simulink model "SensorFaultInj"  (R2013a)
settings: Solver=FixedStepDiscrete  SolverMode=SingleTasking  StartTime=0.0  StopTime=SimLength  FixedStep=SampleTime  RelTol=1e-3
values from neighbouring files (symbols this model uses):
  GlobalSeed = 10    [start_framework07.m]
  SampleTime = 0.01    [start_framework07.m]
  SimLength = 40    [start_framework07.m]
undefined symbols (not defined in the file or in its folder): DiscIntNeverNeededParam
libraries: dspswit3 x48, simulink x32
(part 1 of 9)
settings Model: Creator=Maik  LastModifiedBy=Maik
settings DebuggingCC: AlgebraicLoopMsg=none  UnconnectedOutputMsg=none  BusObjectLabelMismatch=none

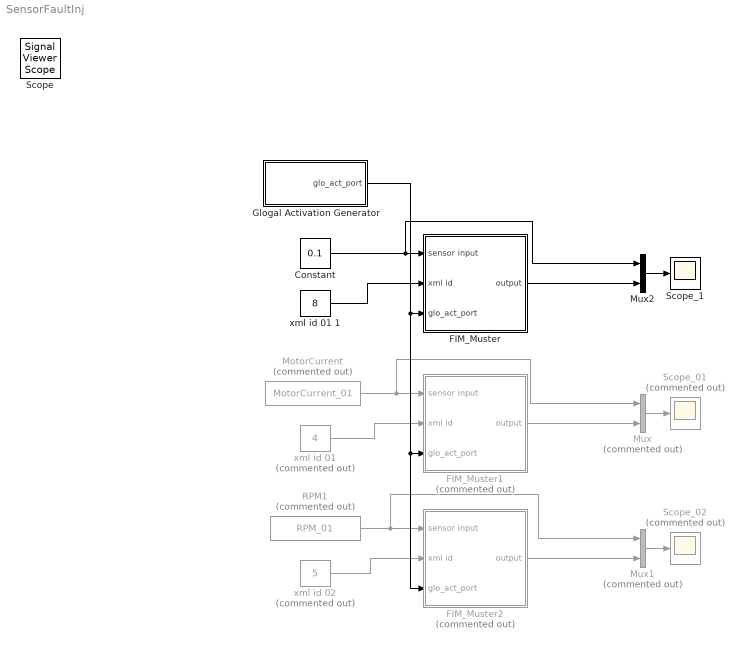
== system SensorFaultInj ==
  Constant : Constant  Value=0.1
  FIM_Muster : Subsystem
  FIM_Muster1 : Subsystem  Commented=on
  FIM_Muster2 : Subsystem  Commented=on
  Glogal Activation Generator : Subsystem  TreatAsAtomicUnit=on
  "MotorCurrent " : FromWorkspace  Commented=on  VariableName=MotorCurrent_01  SampleTime=SampleTime
  Mux : Mux  Commented=on  Inputs=2
  Mux1 : Mux  Commented=on  Inputs=2
  Mux2 : Mux  Inputs=2
  RPM1 : FromWorkspace  Commented=on  VariableName=RPM_01  SampleTime=SampleTime
  Scope_01 : Scope  Commented=on
      settings: YMin=0  YMax=4
  Scope_02 : Scope  Commented=on
      settings: YMin=0  YMax=20000
  Scope_1 : Scope
      settings: TimeRange=40  YMin=0.1  YMax=0.165  SaveName=SensordataEva01  MaxDataPoints=50000
  "xml id 01 " : Constant  Commented=on  Value=4  OutDataTypeStr=single
  xml id 01 1 : Constant  Value=8  OutDataTypeStr=single
  xml id 02 : Constant  Commented=on  Value=5  OutDataTypeStr=single
  Scope : SignalViewerScope  IOType=viewer  RefreshTime=0.035000
  wires:
  "MotorCurrent "/1 -> FIM_Muster1/1(sensor input), Mux/1
  "xml id 01 "/1 -> FIM_Muster1/2(xml id)
  Mux/1 -> Scope_01/1
  FIM_Muster1/1(output) -> Mux/2
  xml id 02/1 -> FIM_Muster2/2(xml id)
  Mux1/1 -> Scope_02/1
  FIM_Muster2/1(output) -> Mux1/2
  RPM1/1 -> FIM_Muster2/1(sensor input), Mux1/1
  Mux2/1 -> Scope_1/1
  FIM_Muster/1(output) -> Mux2/2
  Constant/1 -> Mux2/1, FIM_Muster/1(sensor input)
  xml id 01 1/1 -> FIM_Muster/2(xml id)
  Glogal Activation Generator/1(glo_act_port) -> FIM_Muster2/3(glo_act_port), FIM_Muster1/3(glo_act_port), FIM_Muster/3(glo_act_port)

== system SensorFaultInj/FIM_Muster ==
  sensor input : Inport
  xml id : Inport  Port=2
  glo_act_port : Inport  Port=3
  Fault Injection Modul : Subsystem
  Local Activation Generator : Subsystem
  Parser Modul : Subsystem
  logger : Subsystem
  output : Outport
  wires:
  Parser Modul/1(schedule_port) -> Local Activation Generator/1(schedule_port), Fault Injection Modul/2(schedule_port)
  Parser Modul/2(occurrnce_port) -> Local Activation Generator/2(occurrence_port)
  Local Activation Generator/1(activation_port) -> Fault Injection Modul/3(activation_port)
  Fault Injection Modul/1(Out1) -> logger/2("input "), output/1
  sensor input/1 -> Fault Injection Modul/1(sensor input)
  xml id/1 -> logger/1(xml_id), Parser Modul/1(xml id)
  Parser Modul/3(parameter_port) -> Local Activation Generator/3("param_port "), Fault Injection Modul/4(parameter_port)
  Fault Injection Modul/2("amplitude_port ") -> logger/4("amp_port ")
  Local Activation Generator/2(log_port) -> logger/3("act_port ")
  glo_act_port/1 -> Local Activation Generator/4(glo_act_port)

== system SensorFaultInj/FIM_Muster1 ==
  sensor input : Inport
  xml id : Inport  Port=2
  glo_act_port : Inport  Port=3
  Fault Injection Modul : Subsystem
  Parser Modul : Subsystem
  logger : Subsystem
  occurrence1 : Subsystem
  output : Outport
  wires:
  Parser Modul/1(schedule_port) -> occurrence1/1(schedule_port), Fault Injection Modul/2(schedule_port)
  Parser Modul/2(occurrnce_port) -> occurrence1/2(occurrence_port)
  occurrence1/1(activation_port) -> Fault Injection Modul/3(activation_port)
  Fault Injection Modul/1(Out1) -> logger/2("input "), output/1
  sensor input/1 -> Fault Injection Modul/1(sensor input)
  xml id/1 -> logger/1(xml_id), Parser Modul/1(xml id)
  Parser Modul/3(parameter_port) -> occurrence1/3("param_port "), Fault Injection Modul/4(parameter_port)
  Fault Injection Modul/2("amplitude_port ") -> logger/4("amp_port ")
  occurrence1/2(log_port) -> logger/3("act_port ")
  glo_act_port/1 -> occurrence1/4(glo_act_port)

== system SensorFaultInj/FIM_Muster2 ==
  sensor input : Inport
  xml id : Inport  Port=2
  glo_act_port : Inport  Port=3
  Fault Injection Modul : Subsystem
  Parser Modul : Subsystem
  logger : Subsystem
  occurrence1 : Subsystem
  output : Outport
  wires:
  Parser Modul/1(schedule_port) -> occurrence1/1(schedule_port), Fault Injection Modul/2(schedule_port)
  Parser Modul/2(occurrnce_port) -> occurrence1/2(occurrence_port)
  occurrence1/1(activation_port) -> Fault Injection Modul/3(activation_port)
  Fault Injection Modul/1(Out1) -> logger/2("input "), output/1
  sensor input/1 -> Fault Injection Modul/1(sensor input)
  xml id/1 -> logger/1(xml_id), Parser Modul/1(xml id)
  Parser Modul/3(parameter_port) -> occurrence1/3("param_port "), Fault Injection Modul/4(parameter_port)
  Fault Injection Modul/2("amplitude_port ") -> logger/4("amp_port ")
  occurrence1/2(log_port) -> logger/3("act_port ")
  glo_act_port/1 -> occurrence1/4(glo_act_port)

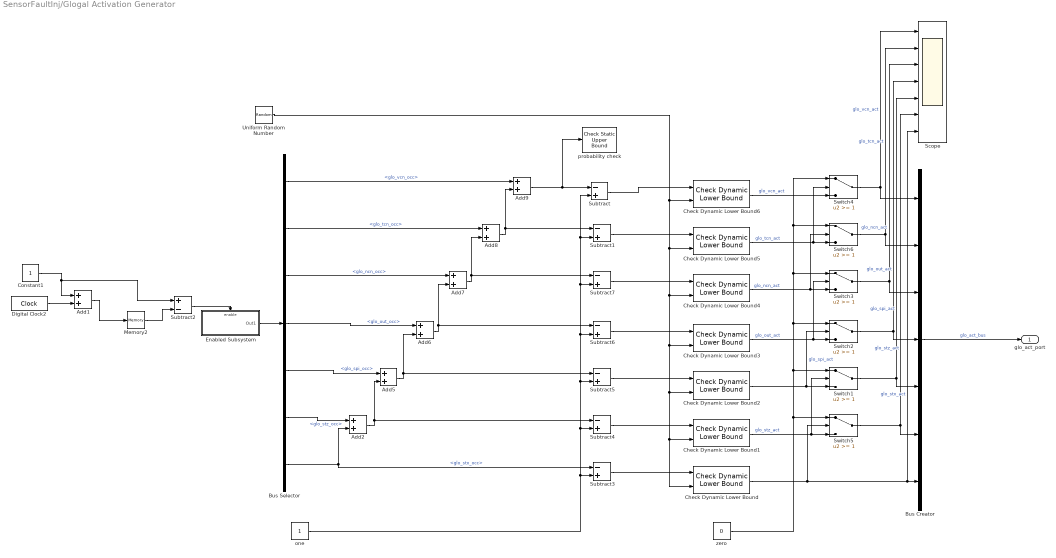
== system SensorFaultInj/Glogal Activation Generator ==
  Add{1..2,5..9} (7 alike) : Sum
  Bus Creator : BusCreator  Inputs=7
  Bus Selector : BusSelector  OutputSignals=glo_vcn_occ,glo_tcn_occ,glo_ncn_occ,glo_out_occ,glo_spi_occ,glo_stz_occ,glo_stx_occ
  Check Dynamic Lower Bound{,1..6} (7 alike) : simulink/Model Verification/Check Dynamic  Lower Bound  Description=min < sig  Enabled=off  stopWhenAssertionFail=off  export=on  icon=graphic
  Constant1 : Constant
  Digital Clock2 : DigitalClock  SampleTime=SampleTime
  Enabled Subsystem : Subsystem  TreatAsAtomicUnit=on
  Memory2 : Memory
  Scope : Scope  NumInputPorts=7
      settings: YMin=-5~-5~-5~-5~-5~-5~-5  YMax=5~5~5~5~5~5~5  SaveName=ScopeData10
  Subtract{,1,3..7} (7 alike) : Sum  Inputs=-+
  Subtract2 : Sum  Inputs=+-
  Switch{1..6} (6 alike) : Switch  Threshold=1
      settings: LockScale=on
  Uniform Random Number : UniformRandomNumber  Seed=GlobalSeed  SampleTime=SampleTime
  one : Constant
  probability check : simulink/Model Verification/Check Static  Upper Bound  Description=u <= 1  max=1  max_included=on  enabled=on  stopWhenAssertionFail=on  export=off  icon=graphic
  zero : Constant  Value=0
  glo_act_port : Outport
  wires:
  Bus Selector/7 -> Subtract3/1, Add2/2  "<glo_stx_occ>"
  Bus Selector/6 -> Add2/1  "<glo_stz_occ>"
  Add5/1 -> Add6/2, Subtract5/1
  Bus Selector/5 -> Add5/1  "<glo_spi_occ>"
  Bus Selector/4 -> Add6/1  "<glo_out_occ>"
  Add6/1 -> Add7/2, Subtract6/1
  Add7/1 -> Add8/2, Subtract7/1
  Bus Selector/3 -> Add7/1  "<glo_ncn_occ>"
  Bus Selector/2 -> Add8/1  "<glo_tcn_occ>"
  Add8/1 -> Add9/2, Subtract1/1
  Bus Selector/1 -> Add9/1  "<glo_vcn_occ>"
  Uniform Random Number/1 -> Check Dynamic Lower Bound/2, Check Dynamic Lower Bound1/2, Check Dynamic Lower Bound2/2, Check Dynamic Lower Bound3/2, Check Dynamic Lower Bound4/2, Check Dynamic Lower Bound5/2, Check Dynamic Lower Bound6/2
  Subtract/1 -> Check Dynamic Lower Bound6/1
  Add9/1 -> probability check/1, Subtract/1
  Subtract1/1 -> Check Dynamic Lower Bound5/1
  Subtract7/1 -> Check Dynamic Lower Bound4/1
  Subtract6/1 -> Check Dynamic Lower Bound3/1
  Subtract5/1 -> Check Dynamic Lower Bound2/1
  Subtract4/1 -> Check Dynamic Lower Bound1/1
  Subtract3/1 -> Check Dynamic Lower Bound/1
  one/1 -> Subtract/2, Subtract1/2, Subtract7/2, Subtract6/2, Subtract5/2, Subtract4/2, Subtract3/2
  Add2/1 -> Subtract4/1, Add5/2
  Check Dynamic Lower Bound/1 -> Switch5/2, Scope/7, Bus Creator/7  "glo_stx_act"
  Switch5/1 -> Bus Creator/6, Scope/6  "glo_stz_act"
  Switch1/1 -> Bus Creator/5, Scope/5  "glo_spi_act"
  Switch2/1 -> Bus Creator/4, Scope/4  "glo_out_act"
  Switch3/1 -> Bus Creator/3, Scope/3  "glo_ncn_act"
  Switch6/1 -> Bus Creator/2, Scope/2  "glo_tcn_act"
  Switch4/1 -> Bus Creator/1, Scope/1  "glo_vcn_act"
  Bus Creator/1 -> glo_act_port/1  "glo_act_bus"
  Check Dynamic Lower Bound1/1 -> Switch1/2, Switch5/3  "glo_stz_act"
  zero/1 -> Switch3/1, Switch6/1, Switch4/1, Switch2/1, Switch1/1, Switch5/1
  Check Dynamic Lower Bound2/1 -> Switch2/2, Switch1/3  "glo_spi_act"
  Check Dynamic Lower Bound3/1 -> Switch3/2, Switch2/3  "glo_out_act"
  Check Dynamic Lower Bound4/1 -> Switch6/2, Switch3/3  "glo_ncn_act"
  Check Dynamic Lower Bound5/1 -> Switch4/2, Switch6/3  "glo_tcn_act"
  Check Dynamic Lower Bound6/1 -> Switch4/3  "glo_vcn_act"
  Digital Clock2/1 -> Add1/2
  Memory2/1 -> Subtract2/2
  Constant1/1 -> Add1/1, Subtract2/1
  Add1/1 -> Memory2/1
  Subtract2/1 -> Enabled Subsystem/Enable
  Enabled Subsystem/1(Out1) -> Bus Selector/1

== system SensorFaultInj/FIM_Muster/Fault Injection Modul ==
  sensor input : Inport
  schedule_port : Inport  Port=2
  activation_port : Inport  Port=3
  parameter_port : Inport  Port=4
  AFI - additive faults injection : Subsystem
  Bus Creator : BusCreator  Inputs=3
  FFI - functional fault injection : Subsystem
  MFI - multiplicative fault injection : Subsystem
  activation bus creator : Subsystem
  schedule bus creator : Subsystem
  schedule bus creator1 : Subsystem
  Out1 : Outport
  "amplitude_port " : Outport  Port=2
  wires:
  MFI - multiplicative fault injection/1(output) -> AFI - additive faults injection/1(input)
  FFI - functional fault injection/1(output) -> Out1/1
  AFI - additive faults injection/1(output) -> FFI - functional fault injection/1(input)
  sensor input/1 -> MFI - multiplicative fault injection/1(In1)
  activation_port/1 -> activation bus creator/1(act_port)
  schedule_port/1 -> schedule bus creator/1(schedule_port)
  schedule bus creator/1(mfi_sched_port) -> MFI - multiplicative fault injection/2(sched_port)
  activation bus creator/1(mfi_act_port) -> MFI - multiplicative fault injection/3(act_port)
  schedule bus creator1/1(mfi_sched_port) -> MFI - multiplicative fault injection/4(param_port)
  schedule bus creator/2(afi_sched_port) -> AFI - additive faults injection/2(sched_bus)
  activation bus creator/2(afi_act_port) -> AFI - additive faults injection/3(act_bus)
  schedule bus creator1/2(afi_sched_port) -> AFI - additive faults injection/4(param_bus)
  schedule bus creator/3(ffi_sched_port) -> FFI - functional fault injection/2(schedule_port)
  schedule bus creator1/3(ffi_sched_port) -> FFI - functional fault injection/3(param_port)
  parameter_port/1 -> schedule bus creator1/1(schedule_port)
  MFI - multiplicative fault injection/2("amplitude_port ") -> Bus Creator/1
  AFI - additive faults injection/2("amplitude_bus ") -> Bus Creator/2
  Bus Creator/1 -> "amplitude_port "/1  "ampl_bus"
  FFI - functional fault injection/2(amplitude_port) -> Bus Creator/3

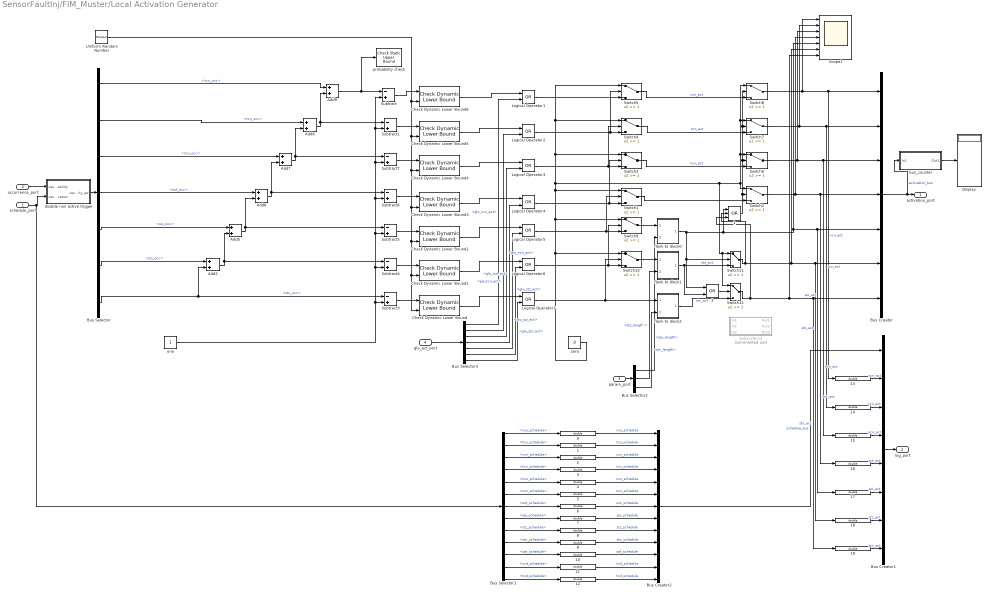
== system SensorFaultInj/FIM_Muster/Local Activation Generator ==
  schedule_port : Inport
  occurrence_port : Inport  Port=2
  "param_port " : Inport  Port=3
  glo_act_port : Inport  Port=4
  " 1" : Logic  Operator=OR  Inputs=3  AllPortsSameDT=off  OutDataTypeStr=boolean
  " 3" : Logic  Operator=OR  AllPortsSameDT=off  OutDataTypeStr=boolean
  {0..19} (20 alike) : DataTypeConversion  OutDataTypeStr=double
  Add{2,5..9} (6 alike) : Sum
  Bus Creator : BusCreator  Inputs=7
  Bus Creator1 : BusCreator  Inputs=8
  Bus Creator2 : BusCreator  Inputs=13
  Bus Selector : BusSelector  OutputSignals=vcn_occ,tcn_occ,ncn_occ,out_occ,spi_occ,stz_occ,stx_occ
  Bus Selector1 : BusSelector  OutputSignals=vco_schedule,tco_schedule,vcn_schedule,tcn_schedule,nco_schedule,ncn_schedule,out_schedule,spi_schedule,stz_schedule,stx_schedule,sat_schedule,ncd_schedule,tcd_schedule
  Bus Selector2 : BusSelector  OutputSignals=parameter_bus.spi_param_bus.spi_length,parameter_bus.stz_length ,parameter_bus.stx_param_bus.stx_length
  Bus Selector3 : BusSelector  OutputSignals=glo_vcn_act,glo_tcn_act,glo_ncn_act,glo_out_act,glo_spi_act,glo_stz_act,glo_stx_act
  Check Dynamic Lower Bound{,1..6} (7 alike) : simulink/Model Verification/Check Dynamic  Lower Bound  Description=min < sig  Enabled=off  stopWhenAssertionFail=off  export=on  icon=graphic
  Display : Display
  Logical Operator{1..7} (7 alike) : Logic  Operator=OR  AllPortsSameDT=off  OutDataTypeStr=boolean
  Scope1 : Scope  NumInputPorts=7
      settings: TimeRange=1  YMin=-1~0~-5~-5~-5~-5~-5  YMax=1~1~5~5~5~5~5  SaveName=ScopeData23  MaxDataPoints=50000
  Subsystem2 : Subsystem  Commented=on
  Subtract{,1,3..7} (7 alike) : Sum  Inputs=-+
  Switch{1..12} (12 alike) : Switch  Threshold=1
      Switch1 settings: LockScale=on
      Switch10 settings: LockScale=on
      Switch5 settings: LockScale=on
      Switch9 settings: LockScale=on
  Uniform Random Number : UniformRandomNumber  Minimum=0  Seed=1  SampleTime=SampleTime
  bus_counter : Subsystem
  disable non active trigger : Subsystem
  flank to dlock0 : Subsystem
  flank to dlock1 : Subsystem
  flank to dlock2 : Subsystem
  one : Constant
  probability check : simulink/Model Verification/Check Static  Upper Bound  Description=u <= 1  max=1  max_included=on  enabled=on  stopWhenAssertionFail=on  export=off  icon=graphic
  zero : Constant  Value=0  OutDataTypeStr=boolean
  activation_port : Outport
  log_port : Outport  Port=2
  wires:
  Bus Selector/7 -> Add2/2, Subtract3/1  "<stx_occ>"
  Bus Selector/6 -> Add2/1  "<stz_occ>"
  Add5/1 -> Add6/2, Subtract5/1
  Bus Selector/5 -> Add5/1  "<spi_occ>"
  Bus Selector/4 -> Add6/1  "<out_occ>"
  Add6/1 -> Add7/2, Subtract6/1
  Add7/1 -> Add8/2, Subtract7/1
  Bus Selector/3 -> Add7/1  "<ncn_occ>"
  Bus Selector/2 -> Add8/1  "<tcn_occ>"
  Add8/1 -> Add9/2, Subtract1/1
  Bus Selector/1 -> Add9/1  "<vcn_occ>"
  Subtract/1 -> Check Dynamic Lower Bound6/1
  Add9/1 -> probability check/1, Subtract/1
  Subtract1/1 -> Check Dynamic Lower Bound5/1
  Subtract7/1 -> Check Dynamic Lower Bound4/1
  Subtract6/1 -> Check Dynamic Lower Bound3/1
  Subtract5/1 -> Check Dynamic Lower Bound2/1
  Subtract4/1 -> Check Dynamic Lower Bound1/1
  Subtract3/1 -> Check Dynamic Lower Bound/1
  one/1 -> Subtract/2, Subtract1/2, Subtract7/2, Subtract6/2, Subtract5/2, Subtract4/2, Subtract3/2
  zero/1 -> Switch1/1, Switch12/1, Switch11/1, Switch2/1, Switch8/1, Switch7/1, Switch6/1, Switch3/1, Switch4/1, Switch5/1, Switch9/1, Switch10/1
  Switch8/1 -> Scope1/1, 13/1, Bus Creator/1  "vcn_act"
  Switch7/1 -> Scope1/2, 14/1, Bus Creator/2  "tcn_act"
  Switch6/1 -> Scope1/3, 15/1, Bus Creator/3  "ncn_act"
  Switch2/1 -> 16/1, Bus Creator/4, Scope1/4  "out_act"
  flank to dlock0/1(block) -> " 1"/1, Scope1/5, 17/1, Bus Creator/5, Switch11/2, " 3"/1  "spi_act"
  Switch11/1 -> " 1"/2, Scope1/6, 18/1, Bus Creator/6  "stz_act"
  Bus Creator/1 -> activation_port/1, bus_counter/1(In1)  "activation_bus"
  occurrence_port/1 -> disable non active trigger/1(vec_probability)
  schedule_port/1 -> Bus Selector1/1, disable non active trigger/2(vec_activation)
  Add2/1 -> Subtract4/1, Add5/2
  Switch12/1 -> " 1"/3, Scope1/7, 19/1, Bus Creator/7  "stx_act"
  disable non active trigger/1(vec_probability_ad) -> Bus Selector/1
  Bus Creator1/1 -> log_port/1
  Bus Selector1/1 -> 0/1  "<vco_schedule>"
  3/1 -> Bus Creator2/4  "tcn_schedule"
  0/1 -> Bus Creator2/1  "vco_schedule"
  4/1 -> Bus Creator2/5  "nco_schedule"
  1/1 -> Bus Creator2/2  "tco_schedule"
  2/1 -> Bus Creator2/3  "vcn_schedule"
  5/1 -> Bus Creator2/6  "ncn_schedule"
  6/1 -> Bus Creator2/7  "out_schedule"
  12/1 -> Bus Creator2/13  "tcd_schedule"
  7/1 -> Bus Creator2/8  "spi_schedule"
  8/1 -> Bus Creator2/9  "stz_schedule"
  9/1 -> Bus Creator2/10  "stx_schedule"
  10/1 -> Bus Creator2/11  "sat_schedule"
  11/1 -> Bus Creator2/12  "ncd_schedule"
  Bus Selector1/2 -> 1/1  "<tco_schedule>"
  Bus Selector1/3 -> 2/1  "<vcn_schedule>"
  Bus Selector1/4 -> 3/1  "<tcn_schedule>"
  Bus Selector1/5 -> 4/1  "<nco_schedule>"
  Bus Selector1/6 -> 5/1  "<ncn_schedule>"
  Bus Selector1/7 -> 6/1  "<out_schedule>"
  Bus Selector1/8 -> 7/1  "<spi_schedule>"
  Bus Selector1/9 -> 8/1  "<stz_schedule>"
  Bus Selector1/10 -> 9/1  "<stx_schedule>"
  Bus Selector1/11 -> 10/1  "<sat_schedule>"
  Bus Selector1/12 -> 11/1  "<ncd_schedule>"
  Bus Selector1/13 -> 12/1  "<tcd_schedule>"
  Bus Creator2/1 -> Bus Creator1/1  "schedule_bus"
  13/1 -> Bus Creator1/2  "vcn_act"
  14/1 -> Bus Creator1/3  "tcn_act"
  15/1 -> Bus Creator1/4  "ncn_act"
  16/1 -> Bus Creator1/5  "out_act"
  17/1 -> Bus Creator1/6  "spi_act"
  18/1 -> Bus Creator1/7  "stz_act"
  19/1 -> Bus Creator1/8  "stx_act"
  "param_port "/1 -> Bus Selector2/1
  Bus Selector2/1 -> flank to dlock0/2(delay)  "<spi_length>"
  Bus Selector2/2 -> flank to dlock1/2(delay)  "<stz_length >"
  Bus Selector2/3 -> flank to dlock2/2(delay)  "<stx_length>"
  Logical Operator1/1 -> Switch5/3
  Check Dynamic Lower Bound6/1 -> Logical Operator1/1
  Logical Operator3/1 -> Switch3/3, Switch4/2
  Logical Operator2/1 -> Switch5/2, Switch4/3
  Check Dynamic Lower Bound5/1 -> Logical Operator2/1
  Check Dynamic Lower Bound4/1 -> Logical Operator3/1
  Check Dynamic Lower Bound3/1 -> Logical Operator4/1
  Check Dynamic Lower Bound2/1 -> Logical Operator5/1
  Check Dynamic Lower Bound1/1 -> Logical Operator6/1
  Check Dynamic Lower Bound/1 -> Logical Operator7/1
  glo_act_port/1 -> Bus Selector3/1
  Bus Selector3/7 -> Logical Operator7/2  "<glo_stx_act>"
  Bus Selector3/6 -> Logical Operator6/2  "<glo_stz_act>"
  Bus Selector3/5 -> Logical Operator5/2  "<glo_spi_act>"
  Bus Selector3/4 -> Logical Operator4/2  "<glo_out_act>"
  Bus Selector3/3 -> Logical Operator3/2  "<glo_ncn_act>"
  Bus Selector3/2 -> Logical Operator2/2  "<glo_tcn_act>"
  Bus Selector3/1 -> Logical Operator1/2  "<glo_vcn_act>"
  bus_counter/1(Out1) -> Display/1
  Uniform Random Number/1 -> Check Dynamic Lower Bound4/2, Check Dynamic Lower Bound3/2, Check Dynamic Lower Bound2/2, Check Dynamic Lower Bound1/2, Check Dynamic Lower Bound/2, Check Dynamic Lower Bound5/2, Check Dynamic Lower Bound6/2
  " 1"/1 -> Switch6/2, Switch8/2, Switch7/2, Switch2/2
  Switch3/1 -> Switch6/3  "ncn_act"
  Switch4/1 -> Switch7/3  "tcn_act"
  Switch5/1 -> Switch8/3  "vcn_act"
  Switch1/1 -> Switch2/3
  Logical Operator4/1 -> Switch3/2, Switch1/3
  Logical Operator5/1 -> Switch1/2, Switch9/3
  Logical Operator6/1 -> Switch9/2, Switch10/3
  Logical Operator7/1 -> flank to dlock2/1(flank), Switch10/2
  Switch10/1 -> flank to dlock1/1(flank)
  Switch9/1 -> flank to dlock0/1(flank)
  flank to dlock2/1(block) -> Switch12/3  "stx_act"
  flank to dlock1/1(block) -> " 3"/2, Switch11/3  "stz_act"
  " 3"/1 -> Switch12/2

== system SensorFaultInj/FIM_Muster/Parser Modul ==
  xml id : Inport
  Bus Creator : BusCreator  Inputs=2
  Fault Parameter Parser : Subsystem
  "Occurence Parser " : Subsystem
  "Schedule Parser and Generator " : Subsystem
  activation_vec : Display
  occ_vec : Display
  parameter_vec : Display
  schedule : Scope
      settings: SaveName=ScopeData2
  schedule_port : Outport
  occurrnce_port : Outport  Port=2
  parameter_port : Outport  Port=3
  wires:
  "Occurence Parser "/1(Out1) -> occ_vec/1, occurrnce_port/1
  "Schedule Parser and Generator "/1(Out1) -> schedule/1, activation_vec/1, schedule_port/1
  xml id/1 -> "Schedule Parser and Generator "/1(In1), Fault Parameter Parser/1(In1), Bus Creator/2, "Occurence Parser "/1(In1)  "xml_id"
  Fault Parameter Parser/1(Out1) -> parameter_vec/1, Bus Creator/1  "parameter_bus"
  Bus Creator/1 -> parameter_port/1

== system SensorFaultInj/FIM_Muster/logger ==
  xml_id : Inport
  "input " : Inport  Port=2
  "act_port " : Inport  Port=3
  "amp_port " : Inport  Port=4
  Bus Creator : BusCreator  Inputs=13
  Bus Creator1 : BusCreator  Inputs=13
  Bus Selector : BusSelector  OutputSignals=schedule_bus.vco_schedule,schedule_bus.tco_schedule,vcn_act,tcn_act,schedule_bus.nco_schedule,ncn_act,out_act,spi_act,stz_act,stx_act,schedule_bus.sat_schedule,schedule_bus.ncd_schedule,schedule_bus.tcd_schedule
  Bus Selector1 : BusSelector  OutputSignals=mfi_amp_bus.vco_ampl,mfi_amp_bus.tco_ampl,mfi_amp_bus.vcn_ampl,mfi_amp_bus.tcn_ampl,afi_ampl_bus.nco_ampl,afi_ampl_bus.ncn_ampl,afi_ampl_bus.out_ampl,afi_ampl_bus.spike_ampl,afi_ampl_bus.stz_ampl,afi_ampl_bus.stx_ampl,ffi_ampl_bus.sat_ampl,ffi_ampl_bus.ncd_ampl,ffi_ampl_bus.tcd_ampl
  Constant1 : Constant
  Discrete-Time Integrator : DiscreteIntegrator  SampleTime=SampleTime  ICPrevOutput=DiscIntNeverNeededParam  ICPrevScaledInput=DiscIntNeverNeededParam
  Display : Display
  Display1 : Display
  ex_sfun_logger : S-Function  FunctionName=ex_sfun_logger  EnableBusSupport=off  mask(Legacy Function){SFunctionSpec=single y1 = logger(single u1, double u2, double u3, double u4[], double u5[]), ShowSpec=on}
      mask prompts: ShowSpec "Display function specification"
      mask help:
      | This block allows you to call the legacy functions specified by the following Legacy Code Tool definition:
      | def.SFunctionName = 'ex_sfun_logger';
      | def.OutputFcnSpec = 'single y1 = logger(single u1, double u2, double u3, double u4[], double u5[])';
      | def.HeaderFiles = {'logger.hpp'};
      | def.SourceFiles = {'logger.cpp'};
      | def.Options.language = 'C++';
      mask Help: <p>This block was generated automatically by the Legacy Code Tool. For detailed help on this tool, call<a href="matlab:legacy_code('help')"> legacy_code('help')</a>.</p>
      mask Callback ShowSpec:
      | if strcmp(get_param(gcbh, 'ShowSpec'), 'on')
      |   set_param(gcbh, 'MaskDisplay', sprintf('fprintf(''%s'');', get_param(gcbh, 'SFunctionSpec')));
      | else
      |   set_param(gcbh, 'MaskDisplay', sprintf('fprintf(''%s'');', get_param(gcbh, 'FunctionName')));
      | end
      mask Display: fprintf('single y1 = logger(single u1, double u2, double u3, double u4[], double u5[])');
  wires:
  "act_port "/1 -> Bus Selector/1
  "amp_port "/1 -> Bus Selector1/1
  Bus Selector1/2 -> Bus Creator1/2  "<tco_ampl>"
  Bus Selector1/3 -> Bus Creator1/3  "<vcn_ampl>"
  Bus Selector1/4 -> Bus Creator1/4  "<tcn_ampl>"
  Bus Selector1/6 -> Bus Creator1/6  "<ncn_ampl>"
  Bus Selector1/7 -> Bus Creator1/7  "<out_ampl>"
  Bus Selector1/8 -> Bus Creator1/8  "<spike_ampl>"
  Bus Selector1/1 -> Bus Creator1/1  "<vco_ampl>"
  Bus Selector1/5 -> Bus Creator1/5  "<nco_ampl>"
  Bus Selector1/9 -> Bus Creator1/9  "<stz_ampl>"
  Bus Selector1/10 -> Bus Creator1/10  "<stx_ampl>"
  Bus Selector1/13 -> Bus Creator1/13  "<tcd_ampl>"
  Bus Selector1/12 -> Bus Creator1/12  "<ncd_ampl>"
  Bus Selector1/11 -> Bus Creator1/11  "<sat_ampl>"
  Bus Creator/1 -> Display/1, ex_sfun_logger/4
  Bus Creator1/1 -> ex_sfun_logger/5, Display1/1
  xml_id/1 -> ex_sfun_logger/1
  Constant1/1 -> Discrete-Time Integrator/1
  Bus Selector/11 -> Bus Creator/11  "<sat_schedule>"
  Bus Selector/12 -> Bus Creator/12  "<ncd_schedule>"
  Bus Selector/13 -> Bus Creator/13  "<tcd_schedule>"
  Bus Selector/3 -> Bus Creator/3  "<vcn_act>"
  Bus Selector/4 -> Bus Creator/4  "<tcn_act>"
  Bus Selector/5 -> Bus Creator/5  "<nco_schedule>"
  Bus Selector/6 -> Bus Creator/6  "<ncn_act>"
  Bus Selector/8 -> Bus Creator/8  "<spi_act>"
  Bus Selector/10 -> Bus Creator/10  "<stx_act>"
  Bus Selector/9 -> Bus Creator/9  "<stz_act>"
  Bus Selector/7 -> Bus Creator/7  "<out_act>"
  Bus Selector/1 -> Bus Creator/1  "<vco_schedule>"
  Bus Selector/2 -> Bus Creator/2  "<tco_schedule>"
  "input "/1 -> ex_sfun_logger/3
  Discrete-Time Integrator/1 -> ex_sfun_logger/2

== system SensorFaultInj/FIM_Muster1/Fault Injection Modul ==
  sensor input : Inport
  schedule_port : Inport  Port=2
  activation_port : Inport  Port=3
  parameter_port : Inport  Port=4
  AFI - additive faults injection : Subsystem
  Bus Creator : BusCreator  Inputs=3
  FFI - functional fault injection : Subsystem
  MFI - multiplicative fault injection : Subsystem
  activation bus creator : Subsystem
  schedule bus creator : Subsystem
  schedule bus creator1 : Subsystem
  Out1 : Outport
  "amplitude_port " : Outport  Port=2
  wires:
  MFI - multiplicative fault injection/1(output) -> AFI - additive faults injection/1(input)
  FFI - functional fault injection/1(output) -> Out1/1
  AFI - additive faults injection/1(output) -> FFI - functional fault injection/1(input)
  sensor input/1 -> MFI - multiplicative fault injection/1(In1)
  activation_port/1 -> activation bus creator/1(act_port)
  schedule_port/1 -> schedule bus creator/1(schedule_port)
  schedule bus creator/1(mfi_sched_port) -> MFI - multiplicative fault injection/2(sched_port)
  activation bus creator/1(mfi_act_port) -> MFI - multiplicative fault injection/3(act_port)
  schedule bus creator1/1(mfi_sched_port) -> MFI - multiplicative fault injection/4(param_port)
  schedule bus creator/2(afi_sched_port) -> AFI - additive faults injection/2(sched_bus)
  activation bus creator/2(afi_act_port) -> AFI - additive faults injection/3(act_bus)
  schedule bus creator1/2(afi_sched_port) -> AFI - additive faults injection/4(param_bus)
  schedule bus creator/3(ffi_sched_port) -> FFI - functional fault injection/2(schedule_port)
  schedule bus creator1/3(ffi_sched_port) -> FFI - functional fault injection/3(param_port)
  parameter_port/1 -> schedule bus creator1/1(schedule_port)
  MFI - multiplicative fault injection/2("amplitude_port ") -> Bus Creator/1
  AFI - additive faults injection/2("amplitude_bus ") -> Bus Creator/2
  Bus Creator/1 -> "amplitude_port "/1  "ampl_bus"
  FFI - functional fault injection/2(amplitude_port) -> Bus Creator/3

== system SensorFaultInj/FIM_Muster1/Parser Modul ==
  xml id : Inport
  Bus Creator : BusCreator  Inputs=2
  activation_vec : Display
  occ_vec : Display
  "occurence parser " : Subsystem
  parameter parser : Subsystem
  parameter_vec : Display
  schedule : Scope
      settings: SaveName=ScopeData2
  "schedule once per sample step " : Subsystem
  schedule_port : Outport
  occurrnce_port : Outport  Port=2
  parameter_port : Outport  Port=3
  wires:
  "occurence parser "/1(Out1) -> occ_vec/1, occurrnce_port/1
  "schedule once per sample step "/1(Out1) -> schedule/1, activation_vec/1, schedule_port/1
  xml id/1 -> "schedule once per sample step "/1(In1), parameter parser/1(In1), Bus Creator/2, "occurence parser "/1(In1)  "xml_id"
  parameter parser/1(Out1) -> parameter_vec/1, Bus Creator/1  "parameter_bus"
  Bus Creator/1 -> parameter_port/1

== system SensorFaultInj/FIM_Muster1/logger ==
  xml_id : Inport
  "input " : Inport  Port=2
  "act_port " : Inport  Port=3
  "amp_port " : Inport  Port=4
  Bus Creator : BusCreator  Inputs=13
  Bus Creator1 : BusCreator  Inputs=13
  Bus Selector : BusSelector  OutputSignals=schedule_bus.vco_schedule,schedule_bus.tco_schedule,vcn_act,tcn_act,schedule_bus.nco_schedule,ncn_act,out_act,spi_act,stz_act,stx_act,schedule_bus.sat_schedule,schedule_bus.ncd_schedule,schedule_bus.tcd_schedule
  Bus Selector1 : BusSelector  OutputSignals=mfi_amp_bus.vco_ampl,mfi_amp_bus.tco_ampl,mfi_amp_bus.vcn_ampl,mfi_amp_bus.tcn_ampl,afi_ampl_bus.nco_ampl,afi_ampl_bus.ncn_ampl,afi_ampl_bus.out_ampl,afi_ampl_bus.spike_ampl,afi_ampl_bus.stz_ampl,afi_ampl_bus.stx_ampl,ffi_ampl_bus.sat_ampl,ffi_ampl_bus.ncd_ampl,ffi_ampl_bus.tcd_ampl
  Constant1 : Constant
  Discrete-Time Integrator : DiscreteIntegrator  SampleTime=SampleTime  ICPrevOutput=DiscIntNeverNeededParam  ICPrevScaledInput=DiscIntNeverNeededParam
  Display : Display
  Display1 : Display
  ex_sfun_logger : S-Function  FunctionName=ex_sfun_logger  EnableBusSupport=off  mask(Legacy Function){SFunctionSpec=single y1 = logger(single u1, double u2, double u3, double u4[], double u5[]), ShowSpec=on}
      mask prompts: ShowSpec "Display function specification"
      mask help:
      | This block allows you to call the legacy functions specified by the following Legacy Code Tool definition:
      | def.SFunctionName = 'ex_sfun_logger';
      | def.OutputFcnSpec = 'single y1 = logger(single u1, double u2, double u3, double u4[], double u5[])';
      | def.HeaderFiles = {'logger.hpp'};
      | def.SourceFiles = {'logger.cpp'};
      | def.Options.language = 'C++';
      mask Help: <p>This block was generated automatically by the Legacy Code Tool. For detailed help on this tool, call<a href="matlab:legacy_code('help')"> legacy_code('help')</a>.</p>
      mask Callback ShowSpec:
      | if strcmp(get_param(gcbh, 'ShowSpec'), 'on')
      |   set_param(gcbh, 'MaskDisplay', sprintf('fprintf(''%s'');', get_param(gcbh, 'SFunctionSpec')));
      | else
      |   set_param(gcbh, 'MaskDisplay', sprintf('fprintf(''%s'');', get_param(gcbh, 'FunctionName')));
      | end
      mask Display: fprintf('single y1 = logger(single u1, double u2, double u3, double u4[], double u5[])');
  wires:
  "act_port "/1 -> Bus Selector/1
  "amp_port "/1 -> Bus Selector1/1
  Bus Selector1/2 -> Bus Creator1/2  "<tco_ampl>"
  Bus Selector1/3 -> Bus Creator1/3  "<vcn_ampl>"
  Bus Selector1/4 -> Bus Creator1/4  "<tcn_ampl>"
  Bus Selector1/6 -> Bus Creator1/6  "<ncn_ampl>"
  Bus Selector1/7 -> Bus Creator1/7  "<out_ampl>"
  Bus Selector1/8 -> Bus Creator1/8  "<spike_ampl>"
  Bus Selector1/1 -> Bus Creator1/1  "<vco_ampl>"
  Bus Selector1/5 -> Bus Creator1/5  "<nco_ampl>"
  Bus Selector1/9 -> Bus Creator1/9  "<stz_ampl>"
  Bus Selector1/10 -> Bus Creator1/10  "<stx_ampl>"
  Bus Selector1/13 -> Bus Creator1/13  "<tcd_ampl>"
  Bus Selector1/12 -> Bus Creator1/12  "<ncd_ampl>"
  Bus Selector1/11 -> Bus Creator1/11  "<sat_ampl>"
  Bus Creator/1 -> Display/1, ex_sfun_logger/4
  Bus Creator1/1 -> ex_sfun_logger/5, Display1/1
  xml_id/1 -> ex_sfun_logger/1
  Constant1/1 -> Discrete-Time Integrator/1
  Bus Selector/11 -> Bus Creator/11  "<sat_schedule>"
  Bus Selector/12 -> Bus Creator/12  "<ncd_schedule>"
  Bus Selector/13 -> Bus Creator/13  "<tcd_schedule>"
  Bus Selector/3 -> Bus Creator/3  "<vcn_act>"
  Bus Selector/4 -> Bus Creator/4  "<tcn_act>"
  Bus Selector/5 -> Bus Creator/5  "<nco_schedule>"
  Bus Selector/6 -> Bus Creator/6  "<ncn_act>"
  Bus Selector/8 -> Bus Creator/8  "<spi_act>"
  Bus Selector/10 -> Bus Creator/10  "<stx_act>"
  Bus Selector/9 -> Bus Creator/9  "<stz_act>"
  Bus Selector/7 -> Bus Creator/7  "<out_act>"
  Bus Selector/1 -> Bus Creator/1  "<vco_schedule>"
  Bus Selector/2 -> Bus Creator/2  "<tco_schedule>"
  "input "/1 -> ex_sfun_logger/3
  Discrete-Time Integrator/1 -> ex_sfun_logger/2

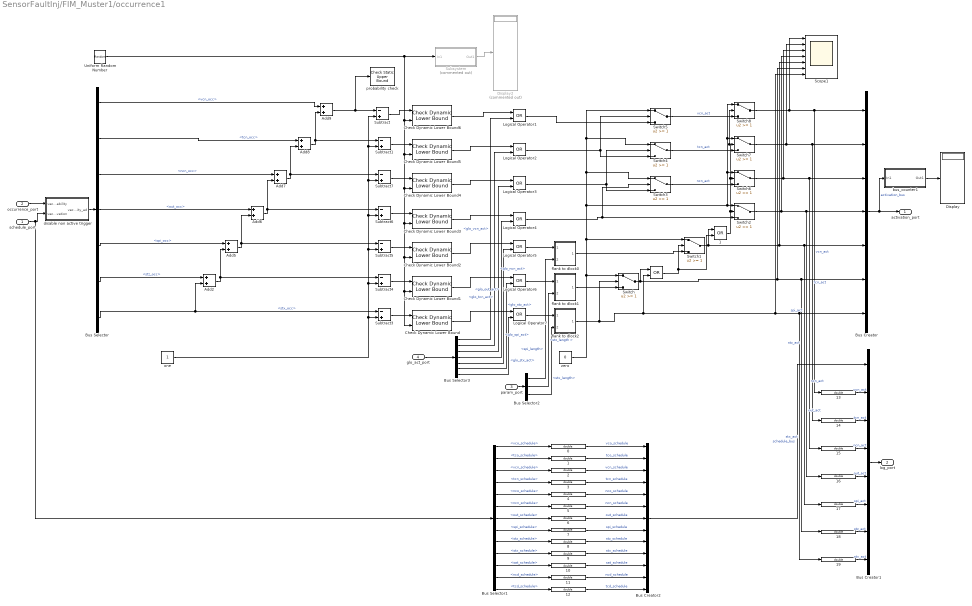
== system SensorFaultInj/FIM_Muster1/occurrence1 ==
  schedule_port : Inport
  occurrence_port : Inport  Port=2
  "param_port " : Inport  Port=3
  glo_act_port : Inport  Port=4
  " " : Logic  Operator=OR  AllPortsSameDT=off  OutDataTypeStr=boolean
  " 1" : Logic  Operator=OR  AllPortsSameDT=off  OutDataTypeStr=boolean
  {0..19} (20 alike) : DataTypeConversion  OutDataTypeStr=double
  Add{2,5..9} (6 alike) : Sum
  Bus Creator : BusCreator  Inputs=7
  Bus Creator1 : BusCreator  Inputs=8
  Bus Creator2 : BusCreator  Inputs=13
  Bus Selector : BusSelector  OutputSignals=vcn_occ,tcn_occ,ncn_occ,out_occ,spi_occ,stz_occ,stx_occ
  Bus Selector1 : BusSelector  OutputSignals=vco_schedule,tco_schedule,vcn_schedule,tcn_schedule,nco_schedule,ncn_schedule,out_schedule,spi_schedule,stz_schedule,stx_schedule,sat_schedule,ncd_schedule,tcd_schedule
  Bus Selector2 : BusSelector  OutputSignals=parameter_bus.spi_param_bus.spi_length,parameter_bus.stz_length ,parameter_bus.stx_param_bus.stx_length
  Bus Selector3 : BusSelector  OutputSignals=glo_vcn_act,glo_tcn_act,glo_ncn_act,glo_out_act,glo_spi_act,glo_stz_act,glo_stx_act
  Check Dynamic Lower Bound{,1..6} (7 alike) : simulink/Model Verification/Check Dynamic  Lower Bound  Description=min < sig  Enabled=off  stopWhenAssertionFail=off  export=on  icon=graphic
  Display : Display
  Display2 : Display  Commented=on
  Logical Operator{1..7} (7 alike) : Logic  Operator=OR  AllPortsSameDT=off  OutDataTypeStr=boolean
  Scope1 : Scope  NumInputPorts=7
      settings: TimeRange=1  YMin=-1~0~-5~-5~-5~-5~-5  YMax=1~1~5~5~5~5~5  SaveName=ScopeData23  MaxDataPoints=50000
  Subsystem : Subsystem  Commented=on
  Subtract{,1,3..7} (7 alike) : Sum  Inputs=-+
  Switch{,1..8} (9 alike) : Switch  Threshold=1
      Switch5 settings: LockScale=on
  Uniform Random Number : UniformRandomNumber  Minimum=0  Seed=1  SampleTime=SampleTime
  bus_counter1 : Subsystem
  disable non active trigger : Subsystem
  flank to dlock0 : Subsystem
  flank to dlock1 : Subsystem
  flank to dlock2 : Subsystem
  one : Constant
  probability check : simulink/Model Verification/Check Static  Upper Bound  Description=u <= 1  max=1  max_included=on  enabled=on  stopWhenAssertionFail=on  export=off  icon=graphic
  zero : Constant  Value=0  OutDataTypeStr=boolean
  activation_port : Outport
  log_port : Outport  Port=2
  wires:
  Bus Selector/7 -> Add2/2, Subtract3/1  "<stx_occ>"
  Bus Selector/6 -> Add2/1  "<stz_occ>"
  Add5/1 -> Add6/2, Subtract5/1
  Bus Selector/5 -> Add5/1  "<spi_occ>"
  Bus Selector/4 -> Add6/1  "<out_occ>"
  Add6/1 -> Add7/2, Subtract6/1
  Add7/1 -> Add8/2, Subtract7/1
  Bus Selector/3 -> Add7/1  "<ncn_occ>"
  Bus Selector/2 -> Add8/1  "<tcn_occ>"
  Add8/1 -> Add9/2, Subtract1/1
  Bus Selector/1 -> Add9/1  "<vcn_occ>"
  Subtract/1 -> Check Dynamic Lower Bound6/1
  Add9/1 -> probability check/1, Subtract/1
  Subtract1/1 -> Check Dynamic Lower Bound5/1
  Subtract7/1 -> Check Dynamic Lower Bound4/1
  Subtract6/1 -> Check Dynamic Lower Bound3/1
  Subtract5/1 -> Check Dynamic Lower Bound2/1
  Subtract4/1 -> Check Dynamic Lower Bound1/1
  Subtract3/1 -> Check Dynamic Lower Bound/1
  one/1 -> Subtract/2, Subtract1/2, Subtract7/2, Subtract6/2, Subtract5/2, Subtract4/2, Subtract3/2
  zero/1 -> Switch1/1, Switch8/1, Switch7/1, Switch6/1, Switch2/1, Switch5/1, Switch4/1, Switch3/1, Switch/1
  flank to dlock0/1(block) -> Switch1/3
  Switch8/1 -> Scope1/1, 13/1, Bus Creator/1  "vcn_act"
  Switch7/1 -> Scope1/2, 14/1, Bus Creator/2  "tcn_act"
  Switch6/1 -> Scope1/3, 15/1, Bus Creator/3  "ncn_act"
  Switch2/1 -> 16/1, Bus Creator/4, Scope1/4  "out_act"
  Switch1/1 -> " 1"/1, Scope1/5, 17/1, Bus Creator/5  "spi_act"
  Switch/1 -> 18/1, Bus Creator/6, Scope1/6, " "/1  "stz_act"
  Bus Creator/1 -> activation_port/1, bus_counter1/1(In1)  "activation_bus"
  occurrence_port/1 -> disable non active trigger/1(vec_probability)
  schedule_port/1 -> Bus Selector1/1, disable non active trigger/2(vec_activation)
  Add2/1 -> Subtract4/1, Add5/2
  flank to dlock2/1(block) -> 19/1, Bus Creator/7, Scope1/7, " "/2, Switch/2  "stx_act"
  flank to dlock1/1(block) -> Switch/3
  disable non active trigger/1(vec_probability_ad) -> Bus Selector/1
  Bus Creator1/1 -> log_port/1
  Bus Selector1/1 -> 0/1  "<vco_schedule>"
  3/1 -> Bus Creator2/4  "tcn_schedule"
  0/1 -> Bus Creator2/1  "vco_schedule"
  4/1 -> Bus Creator2/5  "nco_schedule"
  1/1 -> Bus Creator2/2  "tco_schedule"
  2/1 -> Bus Creator2/3  "vcn_schedule"
  5/1 -> Bus Creator2/6  "ncn_schedule"
  6/1 -> Bus Creator2/7  "out_schedule"
  12/1 -> Bus Creator2/13  "tcd_schedule"
  7/1 -> Bus Creator2/8  "spi_schedule"
  8/1 -> Bus Creator2/9  "stz_schedule"
  9/1 -> Bus Creator2/10  "stx_schedule"
  10/1 -> Bus Creator2/11  "sat_schedule"
  11/1 -> Bus Creator2/12  "ncd_schedule"
  Bus Selector1/2 -> 1/1  "<tco_schedule>"
  Bus Selector1/3 -> 2/1  "<vcn_schedule>"
  Bus Selector1/4 -> 3/1  "<tcn_schedule>"
  Bus Selector1/5 -> 4/1  "<nco_schedule>"
  Bus Selector1/6 -> 5/1  "<ncn_schedule>"
  Bus Selector1/7 -> 6/1  "<out_schedule>"
  Bus Selector1/8 -> 7/1  "<spi_schedule>"
  Bus Selector1/9 -> 8/1  "<stz_schedule>"
  Bus Selector1/10 -> 9/1  "<stx_schedule>"
  Bus Selector1/11 -> 10/1  "<sat_schedule>"
  Bus Selector1/12 -> 11/1  "<ncd_schedule>"
  Bus Selector1/13 -> 12/1  "<tcd_schedule>"
  Bus Creator2/1 -> Bus Creator1/1  "schedule_bus"
  13/1 -> Bus Creator1/2  "vcn_act"
  14/1 -> Bus Creator1/3  "tcn_act"
  15/1 -> Bus Creator1/4  "ncn_act"
  16/1 -> Bus Creator1/5  "out_act"
  17/1 -> Bus Creator1/6  "spi_act"
  18/1 -> Bus Creator1/7  "stz_act"
  19/1 -> Bus Creator1/8  "stx_act"
  "param_port "/1 -> Bus Selector2/1
  Bus Selector2/1 -> flank to dlock0/2(delay)  "<spi_length>"
  Bus Selector2/2 -> flank to dlock1/2(delay)  "<stz_length >"
  Bus Selector2/3 -> flank to dlock2/2(delay)  "<stx_length>"
  Logical Operator1/1 -> Switch5/3
  Check Dynamic Lower Bound6/1 -> Logical Operator1/1
  Logical Operator4/1 -> Switch2/3, Switch3/2
  Logical Operator3/1 -> Switch4/2, Switch3/3
  Logical Operator2/1 -> Switch5/2, Switch4/3
  Logical Operator5/1 -> flank to dlock0/1(flank)
  Logical Operator6/1 -> flank to dlock1/1(flank)
  Logical Operator7/1 -> flank to dlock2/1(flank)
  Check Dynamic Lower Bound5/1 -> Logical Operator2/1
  Check Dynamic Lower Bound4/1 -> Logical Operator3/1
  Check Dynamic Lower Bound3/1 -> Logical Operator4/1
  Check Dynamic Lower Bound2/1 -> Logical Operator5/1
  Check Dynamic Lower Bound1/1 -> Logical Operator6/1
  Check Dynamic Lower Bound/1 -> Logical Operator7/1
  glo_act_port/1 -> Bus Selector3/1
  Bus Selector3/7 -> Logical Operator7/2  "<glo_stx_act>"
  Bus Selector3/6 -> Logical Operator6/2  "<glo_stz_act>"
  Bus Selector3/5 -> Logical Operator5/2  "<glo_spi_act>"
  Bus Selector3/4 -> Logical Operator4/2  "<glo_out_act>"
  Bus Selector3/3 -> Logical Operator3/2  "<glo_ncn_act>"
  Bus Selector3/2 -> Logical Operator2/2  "<glo_tcn_act>"
  Bus Selector3/1 -> Logical Operator1/2  "<glo_vcn_act>"
  bus_counter1/1(Out1) -> Display/1
  Uniform Random Number/1 -> Check Dynamic Lower Bound4/2, Check Dynamic Lower Bound3/2, Check Dynamic Lower Bound2/2, Check Dynamic Lower Bound1/2, Check Dynamic Lower Bound/2, Check Dynamic Lower Bound5/2, Check Dynamic Lower Bound6/2, Subsystem/1(In1)
  " "/1 -> " 1"/2, Switch1/2
  " 1"/1 -> Switch6/2, Switch8/2, Switch7/2, Switch2/2
  Switch3/1 -> Switch6/3  "ncn_act"
  Switch4/1 -> Switch7/3  "tcn_act"
  Switch5/1 -> Switch8/3  "vcn_act"
  Subsystem/1(Out1) -> Display2/1

== system SensorFaultInj/FIM_Muster2/Fault Injection Modul ==
  sensor input : Inport
  schedule_port : Inport  Port=2
  activation_port : Inport  Port=3
  parameter_port : Inport  Port=4
  AFI - additive faults injection : Subsystem
  Bus Creator : BusCreator  Inputs=3
  FFI - functional fault injection : Subsystem
  MFI - multiplicative fault injection : Subsystem
  activation bus creator : Subsystem
  schedule bus creator : Subsystem
  schedule bus creator1 : Subsystem
  Out1 : Outport
  "amplitude_port " : Outport  Port=2
  wires:
  MFI - multiplicative fault injection/1(output) -> AFI - additive faults injection/1(input)
  FFI - functional fault injection/1(output) -> Out1/1
  AFI - additive faults injection/1(output) -> FFI - functional fault injection/1(input)
  sensor input/1 -> MFI - multiplicative fault injection/1(In1)
  activation_port/1 -> activation bus creator/1(act_port)
  schedule_port/1 -> schedule bus creator/1(schedule_port)
  schedule bus creator/1(mfi_sched_port) -> MFI - multiplicative fault injection/2(sched_port)
  activation bus creator/1(mfi_act_port) -> MFI - multiplicative fault injection/3(act_port)
  schedule bus creator1/1(mfi_sched_port) -> MFI - multiplicative fault injection/4(param_port)
  schedule bus creator/2(afi_sched_port) -> AFI - additive faults injection/2(sched_bus)
  activation bus creator/2(afi_act_port) -> AFI - additive faults injection/3(act_bus)
  schedule bus creator1/2(afi_sched_port) -> AFI - additive faults injection/4(param_bus)
  schedule bus creator/3(ffi_sched_port) -> FFI - functional fault injection/2(schedule_port)
  schedule bus creator1/3(ffi_sched_port) -> FFI - functional fault injection/3(param_port)
  parameter_port/1 -> schedule bus creator1/1(schedule_port)
  MFI - multiplicative fault injection/2("amplitude_port ") -> Bus Creator/1
  AFI - additive faults injection/2("amplitude_bus ") -> Bus Creator/2
  Bus Creator/1 -> "amplitude_port "/1  "ampl_bus"
  FFI - functional fault injection/2(amplitude_port) -> Bus Creator/3

== system SensorFaultInj/FIM_Muster2/Parser Modul ==
  xml id : Inport
  Bus Creator : BusCreator  Inputs=2
  activation_vec : Display
  occ_vec : Display
  "occurence parser " : Subsystem
  parameter parser : Subsystem
  parameter_vec : Display
  schedule : Scope
      settings: SaveName=ScopeData2
  "schedule once per sample step " : Subsystem
  schedule_port : Outport
  occurrnce_port : Outport  Port=2
  parameter_port : Outport  Port=3
  wires:
  "occurence parser "/1(Out1) -> occ_vec/1, occurrnce_port/1
  "schedule once per sample step "/1(Out1) -> schedule/1, activation_vec/1, schedule_port/1
  xml id/1 -> "schedule once per sample step "/1(In1), parameter parser/1(In1), Bus Creator/2, "occurence parser "/1(In1)  "xml_id"
  parameter parser/1(Out1) -> parameter_vec/1, Bus Creator/1  "parameter_bus"
  Bus Creator/1 -> parameter_port/1

== system SensorFaultInj/FIM_Muster2/logger ==
  xml_id : Inport
  "input " : Inport  Port=2
  "act_port " : Inport  Port=3
  "amp_port " : Inport  Port=4
  Bus Creator : BusCreator  Inputs=13
  Bus Creator1 : BusCreator  Inputs=13
  Bus Selector : BusSelector  OutputSignals=schedule_bus.vco_schedule,schedule_bus.tco_schedule,vcn_act,tcn_act,schedule_bus.nco_schedule,ncn_act,out_act,spi_act,stz_act,stx_act,schedule_bus.sat_schedule,schedule_bus.ncd_schedule,schedule_bus.tcd_schedule
  Bus Selector1 : BusSelector  OutputSignals=mfi_amp_bus.vco_ampl,mfi_amp_bus.tco_ampl,mfi_amp_bus.vcn_ampl,mfi_amp_bus.tcn_ampl,afi_ampl_bus.nco_ampl,afi_ampl_bus.ncn_ampl,afi_ampl_bus.out_ampl,afi_ampl_bus.spike_ampl,afi_ampl_bus.stz_ampl,afi_ampl_bus.stx_ampl,ffi_ampl_bus.sat_ampl,ffi_ampl_bus.ncd_ampl,ffi_ampl_bus.tcd_ampl
  Constant1 : Constant
  Discrete-Time Integrator : DiscreteIntegrator  SampleTime=SampleTime  ICPrevOutput=DiscIntNeverNeededParam  ICPrevScaledInput=DiscIntNeverNeededParam
  Display : Display
  Display1 : Display
  ex_sfun_logger : S-Function  FunctionName=ex_sfun_logger  EnableBusSupport=off  mask(Legacy Function){SFunctionSpec=single y1 = logger(single u1, double u2, double u3, double u4[], double u5[]), ShowSpec=on}
      mask prompts: ShowSpec "Display function specification"
      mask help:
      | This block allows you to call the legacy functions specified by the following Legacy Code Tool definition:
      | def.SFunctionName = 'ex_sfun_logger';
      | def.OutputFcnSpec = 'single y1 = logger(single u1, double u2, double u3, double u4[], double u5[])';
      | def.HeaderFiles = {'logger.hpp'};
      | def.SourceFiles = {'logger.cpp'};
      | def.Options.language = 'C++';
      mask Help: <p>This block was generated automatically by the Legacy Code Tool. For detailed help on this tool, call<a href="matlab:legacy_code('help')"> legacy_code('help')</a>.</p>
      mask Callback ShowSpec:
      | if strcmp(get_param(gcbh, 'ShowSpec'), 'on')
      |   set_param(gcbh, 'MaskDisplay', sprintf('fprintf(''%s'');', get_param(gcbh, 'SFunctionSpec')));
      | else
      |   set_param(gcbh, 'MaskDisplay', sprintf('fprintf(''%s'');', get_param(gcbh, 'FunctionName')));
      | end
      mask Display: fprintf('single y1 = logger(single u1, double u2, double u3, double u4[], double u5[])');
  wires:
  "act_port "/1 -> Bus Selector/1
  "amp_port "/1 -> Bus Selector1/1
  Bus Selector1/2 -> Bus Creator1/2  "<tco_ampl>"
  Bus Selector1/3 -> Bus Creator1/3  "<vcn_ampl>"
  Bus Selector1/4 -> Bus Creator1/4  "<tcn_ampl>"
  Bus Selector1/6 -> Bus Creator1/6  "<ncn_ampl>"
  Bus Selector1/7 -> Bus Creator1/7  "<out_ampl>"
  Bus Selector1/8 -> Bus Creator1/8  "<spike_ampl>"
  Bus Selector1/1 -> Bus Creator1/1  "<vco_ampl>"
  Bus Selector1/5 -> Bus Creator1/5  "<nco_ampl>"
  Bus Selector1/9 -> Bus Creator1/9  "<stz_ampl>"
  Bus Selector1/10 -> Bus Creator1/10  "<stx_ampl>"
  Bus Selector1/13 -> Bus Creator1/13  "<tcd_ampl>"
  Bus Selector1/12 -> Bus Creator1/12  "<ncd_ampl>"
  Bus Selector1/11 -> Bus Creator1/11  "<sat_ampl>"
  Bus Creator/1 -> Display/1, ex_sfun_logger/4
  Bus Creator1/1 -> ex_sfun_logger/5, Display1/1
  xml_id/1 -> ex_sfun_logger/1
  Constant1/1 -> Discrete-Time Integrator/1
  Bus Selector/11 -> Bus Creator/11  "<sat_schedule>"
  Bus Selector/12 -> Bus Creator/12  "<ncd_schedule>"
  Bus Selector/13 -> Bus Creator/13  "<tcd_schedule>"
  Bus Selector/3 -> Bus Creator/3  "<vcn_act>"
  Bus Selector/4 -> Bus Creator/4  "<tcn_act>"
  Bus Selector/5 -> Bus Creator/5  "<nco_schedule>"
  Bus Selector/6 -> Bus Creator/6  "<ncn_act>"
  Bus Selector/8 -> Bus Creator/8  "<spi_act>"
  Bus Selector/10 -> Bus Creator/10  "<stx_act>"
  Bus Selector/9 -> Bus Creator/9  "<stz_act>"
  Bus Selector/7 -> Bus Creator/7  "<out_act>"
  Bus Selector/1 -> Bus Creator/1  "<vco_schedule>"
  Bus Selector/2 -> Bus Creator/2  "<tco_schedule>"
  "input "/1 -> ex_sfun_logger/3
  Discrete-Time Integrator/1 -> ex_sfun_logger/2
